simulink model "manual_control_new"  (R2023a)
settings: Solver=FixedStepAuto  StartTime=0.0  StopTime=inf  FixedStep=Ts_slk  RelTol=1e-3  EnableMultiTasking=on
undefined symbols (not defined in the file): dev, IMU_w_b_bias, Main, meas_pole, P0_phth, P0_ps, pwm_output0, Q_phth, q_ps, R_phth, r_ps, Rz, Ts_EKF_integr, Ts_EKF_meas, Ts_slk, x0_phth, x0_ps
libraries: px4Sensorslib x4, px4lib x1, sharedtransform x1
(part 1 of 2)
settings Model: ExtModeTrigDuration=10  Creator=ArriGE66  LastModifiedBy=User
settings SolverCC: PositivePriorityOrder=on
settings OptimizationCC: EnhancedBackFolding=on  PassReuseOutputArgsAs=Individual arguments  ZeroExternalMemoryAtStartup=off  ZeroInternalMemoryAtStartup=off  MaxStackSize=64  OptimizeBlockOrder=speed  DifferentSizesBufferReuse=on  OptimizationCustomize=off  EfficientTunableParamExpr=on
settings DebuggingCC: ParameterTunabilityLossMsg=error
settings HardwareCC: ProdBitPerPointer=32  ProdBitPerSizeT=32  ProdBitPerPtrDiffT=32  ProdLargestAtomicInteger=Long  ProdLargestAtomicFloat=Double  ProdWordSize=32  ProdLongLongMode=on  ProdHWDeviceType=ARM Compatible->ARM Cortex
settings SFSimCC: MATLABDynamicMemAlloc=off  SimTargetLang=C++
settings RTWCC: Description=Embedded Coder  SystemTargetFile=ert.tlc  HardwareBoard=PX4 Cube Orange  TLCOptions="-aInlineSetEventsForThisBaseRateFcn=TLC_FALSE -aSuppressMultiTaskScheduler=TLC_FALSE  -aRateBasedStepFcn=0"  TemplateMakefile=ert_default_tmf  Toolchain=GNU Tools for PX4 Autopilots  TargetLang=C++
settings CodeAppCC: ForceParamTrailComments=on  IgnoreCustomStorageClasses=off  OperatorAnnotations=on  SimulinkDataObjDesc=on  SFDataObjDesc=on  InsertBlockDesc=on
settings ERTTargetCC: ExtModeTransport=3  ExtModeStaticAlloc=on  ExtModeStaticAllocSize=1024  ExtModeMexFile=ext_xcp  ExtModeIntrfLevel=Level2 - Open

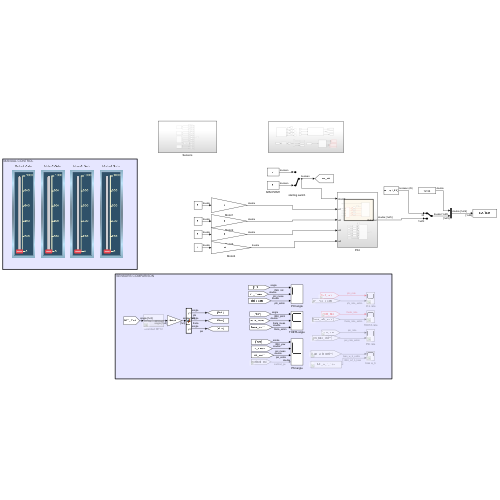
[thumbnail: Simulink's stored preview of the top-level diagram]
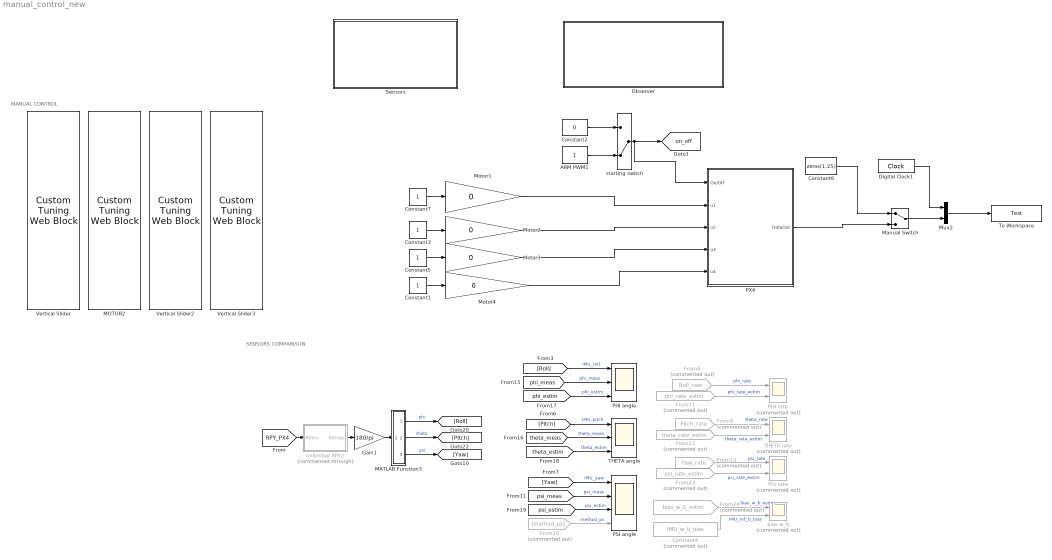
== system manual_control_new ==
  note: SENSORS COMPARISON
  note: MANUAL CONTROL
  ARM PWM1 : Constant  OutDataTypeStr=boolean  SampleTime=Ts_slk
  Constant{1,3,5,7} (4 alike) : Constant  SampleTime=Ts_slk
  Constant2 : Constant  Value=0  OutDataTypeStr=boolean  SampleTime=Ts_slk
  Constant4 : Constant  Commented=on  Value=IMU_w_b_bias
  Constant6 : Constant  Value=zeros(1,25)  OutDataTypeStr=boolean
  Digital Clock1 : DigitalClock  SampleTime=Ts_slk
  From12 : From  Commented=on  GotoTag=Yaw_rate  TagVisibility=global
  From20 : From  Commented=on  GotoTag=method_ps
  From21 : From  Commented=on  GotoTag=phi_rate_estim
  From22 : From  Commented=on  GotoTag=theta_rate_estim
  From23 : From  Commented=on  GotoTag=psi_rate_estim
  From24 : From  Commented=on  GotoTag=bias_w_b_estim
  From8 : From  Commented=on  GotoTag=Roll_rate  TagVisibility=global
  From9 : From  Commented=on  GotoTag=Pitch_rate  TagVisibility=global
  Gain1 : Gain  Gain=180/pi
  MATLAB Function3 : MATLAB Function  TreatAsAtomicUnit=on
  MOTOR2 : CustomTuningWebBlock  ShowInitialText=on  Configuration="{\"components\":[{\"name\":\"LinearScaleComponent\",\"settings\":{\"bounds\":{\"max\":1000,\"min\":0,\"tickInterval\":\"auto\"},\"internalTickHeightScaleFactor\":0.5,\"labelColor\":[255,255,200],\"labelFont\":{\"font\":\"Arial\",\"fontSize\":12},\"labelOffset\":0.05,\"labelTransparency\":1,\"needleImage\":{\"size\":[596,842],\"src\":\"data:image\\/svg+xml;base64,PD94bWwgdmVyc2lvbj0iMS4wIiBlbmNvZGluZz0idXRmLTgiPz4NCjwhLS0gR2VuZXJhdG9yOiBBZG9iZSBJbGx1c3RyYXRvciAyNS4wLjAsIFNWRyBFeHBvcnQgUGx1Zy1JbiAuIFNWRyBWZXJzaW9uOiA2LjAwIEJ1aWxkIDApICAtLT4NCjxzdmcgdmVyc2lvbj0iMS4xIg0KCSBpZD0ic3ZnOCIgeG1sbnM6Y2M9Imh0dHA6Ly9jcmVhdGl2ZWNvbW1vbnMub3JnL25zIyIgeG1sbnM6ZGM9Imh0dHA6Ly9wdXJsLm9yZy9kYy9lbGVtZW50cy8xLjEvIiB4bWxuczppbmtzY2FwZT0iaHR0cDovL3d3dy5pbmtzY2FwZS5vcmcvbmFtZXNw ...(+2420 chars)\",\"srcOrientation\":\"horizontal\"},\"needleOffset\":[0.0642123287671233,-0.8044596912521441],\"needleSize\":{\"height\":0.07668067226890757,\"width\":0.4337797619047619},\"position\":[0.03623949579831933,0.2829861111111111,0.6088789682539683,0.9196428571428571],\"referencePoint\":\"auto\",\"scaleColors\":[],\"scaleColorsSize\":0.2,\"scaleDirection\":\"BT\",\"showLabels\":1,\"showMinorTicks\":0,\"showSpanLine\":1,\"showTicks\":1,\"tickColor\":[252,252,197],\"tickTransparency\":1,\"valueBarColor\":[0,114,189],\"valueBarOffset\":-0.27,\"valueBarSize\":0.1,\"valueBarTransparency\":1}},{\"name\":\"BackgroundImageComponent\",\"settings\":{\"image\":{\"size\":[380,101],\"src\":\"data:image\\/svg+xml;base64,PHN2ZyB4bWxucz0iaHR0cDovL3d3dy53My5vcmcvMjAwMC9zdmciIHhtbG5zOnhsaW5rPSJodHRwOi8vd3d3LnczLm9yZy8xOTk5L3hsaW5rIiB2aWV3Qm94PSIwIDAgMzgwIDEwMSI+PGRlZnM+PHN0eWxlPi5jbHMtMXtmaWxsOiMwMDJiNDI7fS5jbHMtMntmaWxsOiM0MjcwODI7fS5jbHMtM3tmaWxsOnVybCgjcmFkaWFsLWdyYWRpZW50KTt9LmNscy00e2ZpbGw6I2M4YzhjODtzdHJva2U6IzAwMDt9PC9zdHlsZT48cmFkaWFsR3JhZGllbnQgaWQ9InJhZGlhbC1ncmFkaWVudCIgY3g9IjE5MCIgY3k9IjUwLjUiIHI9IjI2OS4yMSIgZ3JhZGllbnRVbml0cz0idXNlclNwYWNlT25Vc2UiPjxzdG9wIG9mZnNldD0iMC4wMSIgc3RvcC1jb2xvcj0iIzNlNGY1OCIvPjxzdG9wIG9mZnNldD0iMC4wNiIgc3RvcC1jb2xvcj0iIzQ0NTc2MSIvPjxzdG9wIG9mZnNldD0iMC4xNSIgc3RvcC1jb2xvcj0iIzU1NmE3NiIvPjxzdG9wIG9mZnNldD0iMC4yNSIgc3RvcC1jb2xvcj0iIzZkODg5NSIvPjxzdG9wIG9mZnNldD0iMC4zOCIgc3RvcC1jb2xvcj0iIzhmYjJjMyIvPjxzdG9wIG9mZnNldD0iMC41MiIgc3RvcC1jb2xvcj0iI2I2ZTRmYSIvPjxzdG9wIG9mZnNldD0iMSIgc3RvcC1jb2xvcj0iIzE1NDY1NyIvPjwvcmFkaWFsR3JhZGllbnQ+PC9kZWZzPjxnIGlkPSJmcmFtZSI+PGcgaWQ9IkxheWVyXzIiIGRhdGEtbmFtZT0iTGF5ZXIgMiI+PGcgaWQ9IkxheWVyXzEtMiIgZGF0YS1uYW1lPSJMYXllciAxLTIiPjxyZWN0IGlkPSJyZWN0MTAzNiIgY2xhc3M9ImNscy0xIiB4PSIxMSIgeT0iMTEiIHdpZHRoPSIzNTgiIGhlaWdodD0iNzkiLz48cGF0aCBpZD0icGF0aDEwMzgiIGNsYXNzPSJjbHMtMiIgZD0iTTgsOFY5M0gzNzJWOFpNMzY5LDkwSDExVjExSDM2OVoiLz48cGF0aCBpZD0icGF0aDEwNDAiIGNsYXNzPSJjbHMtMyIgZD0iTTAsMFYxMDFIMzgwVjBaTTM3Miw5M0g4VjhIMzcyWiIvPjwvZz48L2c+PC9nPjxnIGlkPSJ0cmFjayI+PHBhdGggaWQ9InJlY3QxNjExIiBjbGFzcz0iY2xzLTQiIGQ9Ik0zMy4zNywyNi41OUgzNDYuNjNjNCwwLDcuMjUsMi42LDcuMjUsNS44MWgwYzAsMy4yMS0zLjI1LDUuODItNy4yNSw1LjgySDMzLjM3Yy00LDAtNy4yNS0yLjYxLTcuMjUtNS44MmgwQzI2LjEyLDI5LjE5LDI5LjM3LDI2LjU5LDMzLjM3LDI2LjU5WiIvPjwvZz48L3N2Zz4=\",\"srcOrientation\":\"horizontal\"},\"position\":[0,0,1,1],\"scaleMode\":\"0\"}},{\"name\":\"ForegroundImageComponent\",\"settings\":{\"image\":{\"size\":[0,0],\"src\":\"default\",\"srcOrientation\":[]},\"isForeground\":1,\"position\":[0,0,1,1],\"scaleMode\":\"0\"}}],\"settings\":{\"BindingType\":\"param\",\"aspectRatio\":3.7777777777777777,\"backgroundColor\":[0,0,0,\"1\"],\"backgroundOffset\":0,\"backgroundOpacity\":1,\"fixedAspectRatio\":\"on\",\"foregroundColor\":[252,252,196],\"orientation\":\"vertical\",\"showBackgroundColor\":false,\"value\":0,\"version\":\"R2023a\"},\"type\":\"LinearGauge\"}"
  Manual Switch : ManualSwitch
  Motor{1..4} (4 alike) : Gain  Gain=0
  Mux2 : Mux  Inputs=2
  Observer : Subsystem
  PHI angle : Scope  NumInputPorts=3
  PHI rate : Scope  Commented=on  NumInputPorts=2
  PSI angle : Scope  NumInputPorts=4
  PSI rate : Scope  Commented=on  NumInputPorts=2
  PX4 : Subsystem
  Sensors : Subsystem
  THETA angle : Scope  NumInputPorts=3
  THETA rate : Scope  Commented=on  NumInputPorts=2
  To Workspace : ToWorkspace  VariableName=Test  SampleTime=Ts_slk
      settings: Save2DSignal=2-D array (concatenate along first dimension)
  Vertical Slider : CustomTuningWebBlock  ShowInitialText=on  Configuration="{\"components\":[{\"name\":\"LinearScaleComponent\",\"settings\":{\"bounds\":{\"max\":1000,\"min\":0,\"tickInterval\":\"auto\"},\"internalTickHeightScaleFactor\":0.5,\"labelColor\":[255,255,200],\"labelFont\":{\"font\":\"Arial\",\"fontSize\":12},\"labelOffset\":0.05,\"labelTransparency\":1,\"needleImage\":{\"size\":[596,842],\"src\":\"data:image\\/svg+xml;base64,PD94bWwgdmVyc2lvbj0iMS4wIiBlbmNvZGluZz0idXRmLTgiPz4NCjwhLS0gR2VuZXJhdG9yOiBBZG9iZSBJbGx1c3RyYXRvciAyNS4wLjAsIFNWRyBFeHBvcnQgUGx1Zy1JbiAuIFNWRyBWZXJzaW9uOiA2LjAwIEJ1aWxkIDApICAtLT4NCjxzdmcgdmVyc2lvbj0iMS4xIg0KCSBpZD0ic3ZnOCIgeG1sbnM6Y2M9Imh0dHA6Ly9jcmVhdGl2ZWNvbW1vbnMub3JnL25zIyIgeG1sbnM6ZGM9Imh0dHA6Ly9wdXJsLm9yZy9kYy9lbGVtZW50cy8xLjEvIiB4bWxuczppbmtzY2FwZT0iaHR0cDovL3d3dy5pbmtzY2FwZS5vcmcvbmFtZXNw ...(+2420 chars)\",\"srcOrientation\":\"horizontal\"},\"needleOffset\":[0.0642123287671233,-0.8044596912521441],\"needleSize\":{\"height\":0.07668067226890757,\"width\":0.4337797619047619},\"position\":[0.03623949579831933,0.2829861111111111,0.6088789682539683,0.9196428571428571],\"referencePoint\":\"auto\",\"scaleColors\":[],\"scaleColorsSize\":0.2,\"scaleDirection\":\"BT\",\"showLabels\":1,\"showMinorTicks\":0,\"showSpanLine\":1,\"showTicks\":1,\"tickColor\":[252,252,197],\"tickTransparency\":1,\"valueBarColor\":[0,114,189],\"valueBarOffset\":-0.27,\"valueBarSize\":0.1,\"valueBarTransparency\":1}},{\"name\":\"BackgroundImageComponent\",\"settings\":{\"image\":{\"size\":[380,101],\"src\":\"data:image\\/svg+xml;base64,PHN2ZyB4bWxucz0iaHR0cDovL3d3dy53My5vcmcvMjAwMC9zdmciIHhtbG5zOnhsaW5rPSJodHRwOi8vd3d3LnczLm9yZy8xOTk5L3hsaW5rIiB2aWV3Qm94PSIwIDAgMzgwIDEwMSI+PGRlZnM+PHN0eWxlPi5jbHMtMXtmaWxsOiMwMDJiNDI7fS5jbHMtMntmaWxsOiM0MjcwODI7fS5jbHMtM3tmaWxsOnVybCgjcmFkaWFsLWdyYWRpZW50KTt9LmNscy00e2ZpbGw6I2M4YzhjODtzdHJva2U6IzAwMDt9PC9zdHlsZT48cmFkaWFsR3JhZGllbnQgaWQ9InJhZGlhbC1ncmFkaWVudCIgY3g9IjE5MCIgY3k9IjUwLjUiIHI9IjI2OS4yMSIgZ3JhZGllbnRVbml0cz0idXNlclNwYWNlT25Vc2UiPjxzdG9wIG9mZnNldD0iMC4wMSIgc3RvcC1jb2xvcj0iIzNlNGY1OCIvPjxzdG9wIG9mZnNldD0iMC4wNiIgc3RvcC1jb2xvcj0iIzQ0NTc2MSIvPjxzdG9wIG9mZnNldD0iMC4xNSIgc3RvcC1jb2xvcj0iIzU1NmE3NiIvPjxzdG9wIG9mZnNldD0iMC4yNSIgc3RvcC1jb2xvcj0iIzZkODg5NSIvPjxzdG9wIG9mZnNldD0iMC4zOCIgc3RvcC1jb2xvcj0iIzhmYjJjMyIvPjxzdG9wIG9mZnNldD0iMC41MiIgc3RvcC1jb2xvcj0iI2I2ZTRmYSIvPjxzdG9wIG9mZnNldD0iMSIgc3RvcC1jb2xvcj0iIzE1NDY1NyIvPjwvcmFkaWFsR3JhZGllbnQ+PC9kZWZzPjxnIGlkPSJmcmFtZSI+PGcgaWQ9IkxheWVyXzIiIGRhdGEtbmFtZT0iTGF5ZXIgMiI+PGcgaWQ9IkxheWVyXzEtMiIgZGF0YS1uYW1lPSJMYXllciAxLTIiPjxyZWN0IGlkPSJyZWN0MTAzNiIgY2xhc3M9ImNscy0xIiB4PSIxMSIgeT0iMTEiIHdpZHRoPSIzNTgiIGhlaWdodD0iNzkiLz48cGF0aCBpZD0icGF0aDEwMzgiIGNsYXNzPSJjbHMtMiIgZD0iTTgsOFY5M0gzNzJWOFpNMzY5LDkwSDExVjExSDM2OVoiLz48cGF0aCBpZD0icGF0aDEwNDAiIGNsYXNzPSJjbHMtMyIgZD0iTTAsMFYxMDFIMzgwVjBaTTM3Miw5M0g4VjhIMzcyWiIvPjwvZz48L2c+PC9nPjxnIGlkPSJ0cmFjayI+PHBhdGggaWQ9InJlY3QxNjExIiBjbGFzcz0iY2xzLTQiIGQ9Ik0zMy4zNywyNi41OUgzNDYuNjNjNCwwLDcuMjUsMi42LDcuMjUsNS44MWgwYzAsMy4yMS0zLjI1LDUuODItNy4yNSw1LjgySDMzLjM3Yy00LDAtNy4yNS0yLjYxLTcuMjUtNS44MmgwQzI2LjEyLDI5LjE5LDI5LjM3LDI2LjU5LDMzLjM3LDI2LjU5WiIvPjwvZz48L3N2Zz4=\",\"srcOrientation\":\"horizontal\"},\"position\":[0,0,1,1],\"scaleMode\":\"0\"}},{\"name\":\"ForegroundImageComponent\",\"settings\":{\"image\":{\"size\":[0,0],\"src\":\"default\",\"srcOrientation\":[]},\"isForeground\":1,\"position\":[0,0,1,1],\"scaleMode\":\"0\"}}],\"settings\":{\"BindingType\":\"param\",\"aspectRatio\":3.7777777777777777,\"backgroundColor\":[0,0,0,\"1\"],\"backgroundOffset\":0,\"backgroundOpacity\":1,\"fixedAspectRatio\":\"on\",\"foregroundColor\":[252,252,196],\"orientation\":\"vertical\",\"showBackgroundColor\":false,\"value\":0,\"version\":\"R2023a\"},\"type\":\"LinearGauge\"}"
  Vertical Slider2 : CustomTuningWebBlock  ShowInitialText=on  Configuration="{\"components\":[{\"name\":\"LinearScaleComponent\",\"settings\":{\"bounds\":{\"max\":1000,\"min\":0,\"tickInterval\":\"auto\"},\"internalTickHeightScaleFactor\":0.5,\"labelColor\":[255,255,200],\"labelFont\":{\"font\":\"Arial\",\"fontSize\":12},\"labelOffset\":0.05,\"labelTransparency\":1,\"needleImage\":{\"size\":[596,842],\"src\":\"data:image\\/svg+xml;base64,PD94bWwgdmVyc2lvbj0iMS4wIiBlbmNvZGluZz0idXRmLTgiPz4NCjwhLS0gR2VuZXJhdG9yOiBBZG9iZSBJbGx1c3RyYXRvciAyNS4wLjAsIFNWRyBFeHBvcnQgUGx1Zy1JbiAuIFNWRyBWZXJzaW9uOiA2LjAwIEJ1aWxkIDApICAtLT4NCjxzdmcgdmVyc2lvbj0iMS4xIg0KCSBpZD0ic3ZnOCIgeG1sbnM6Y2M9Imh0dHA6Ly9jcmVhdGl2ZWNvbW1vbnMub3JnL25zIyIgeG1sbnM6ZGM9Imh0dHA6Ly9wdXJsLm9yZy9kYy9lbGVtZW50cy8xLjEvIiB4bWxuczppbmtzY2FwZT0iaHR0cDovL3d3dy5pbmtzY2FwZS5vcmcvbmFtZXNw ...(+2420 chars)\",\"srcOrientation\":\"horizontal\"},\"needleOffset\":[0.0642123287671233,-0.8044596912521441],\"needleSize\":{\"height\":0.07668067226890757,\"width\":0.4337797619047619},\"position\":[0.03623949579831933,0.2829861111111111,0.6088789682539683,0.9196428571428571],\"referencePoint\":\"auto\",\"scaleColors\":[],\"scaleColorsSize\":0.2,\"scaleDirection\":\"BT\",\"showLabels\":1,\"showMinorTicks\":0,\"showSpanLine\":1,\"showTicks\":1,\"tickColor\":[252,252,197],\"tickTransparency\":1,\"valueBarColor\":[0,114,189],\"valueBarOffset\":-0.27,\"valueBarSize\":0.1,\"valueBarTransparency\":1}},{\"name\":\"BackgroundImageComponent\",\"settings\":{\"image\":{\"size\":[380,101],\"src\":\"data:image\\/svg+xml;base64,PHN2ZyB4bWxucz0iaHR0cDovL3d3dy53My5vcmcvMjAwMC9zdmciIHhtbG5zOnhsaW5rPSJodHRwOi8vd3d3LnczLm9yZy8xOTk5L3hsaW5rIiB2aWV3Qm94PSIwIDAgMzgwIDEwMSI+PGRlZnM+PHN0eWxlPi5jbHMtMXtmaWxsOiMwMDJiNDI7fS5jbHMtMntmaWxsOiM0MjcwODI7fS5jbHMtM3tmaWxsOnVybCgjcmFkaWFsLWdyYWRpZW50KTt9LmNscy00e2ZpbGw6I2M4YzhjODtzdHJva2U6IzAwMDt9PC9zdHlsZT48cmFkaWFsR3JhZGllbnQgaWQ9InJhZGlhbC1ncmFkaWVudCIgY3g9IjE5MCIgY3k9IjUwLjUiIHI9IjI2OS4yMSIgZ3JhZGllbnRVbml0cz0idXNlclNwYWNlT25Vc2UiPjxzdG9wIG9mZnNldD0iMC4wMSIgc3RvcC1jb2xvcj0iIzNlNGY1OCIvPjxzdG9wIG9mZnNldD0iMC4wNiIgc3RvcC1jb2xvcj0iIzQ0NTc2MSIvPjxzdG9wIG9mZnNldD0iMC4xNSIgc3RvcC1jb2xvcj0iIzU1NmE3NiIvPjxzdG9wIG9mZnNldD0iMC4yNSIgc3RvcC1jb2xvcj0iIzZkODg5NSIvPjxzdG9wIG9mZnNldD0iMC4zOCIgc3RvcC1jb2xvcj0iIzhmYjJjMyIvPjxzdG9wIG9mZnNldD0iMC41MiIgc3RvcC1jb2xvcj0iI2I2ZTRmYSIvPjxzdG9wIG9mZnNldD0iMSIgc3RvcC1jb2xvcj0iIzE1NDY1NyIvPjwvcmFkaWFsR3JhZGllbnQ+PC9kZWZzPjxnIGlkPSJmcmFtZSI+PGcgaWQ9IkxheWVyXzIiIGRhdGEtbmFtZT0iTGF5ZXIgMiI+PGcgaWQ9IkxheWVyXzEtMiIgZGF0YS1uYW1lPSJMYXllciAxLTIiPjxyZWN0IGlkPSJyZWN0MTAzNiIgY2xhc3M9ImNscy0xIiB4PSIxMSIgeT0iMTEiIHdpZHRoPSIzNTgiIGhlaWdodD0iNzkiLz48cGF0aCBpZD0icGF0aDEwMzgiIGNsYXNzPSJjbHMtMiIgZD0iTTgsOFY5M0gzNzJWOFpNMzY5LDkwSDExVjExSDM2OVoiLz48cGF0aCBpZD0icGF0aDEwNDAiIGNsYXNzPSJjbHMtMyIgZD0iTTAsMFYxMDFIMzgwVjBaTTM3Miw5M0g4VjhIMzcyWiIvPjwvZz48L2c+PC9nPjxnIGlkPSJ0cmFjayI+PHBhdGggaWQ9InJlY3QxNjExIiBjbGFzcz0iY2xzLTQiIGQ9Ik0zMy4zNywyNi41OUgzNDYuNjNjNCwwLDcuMjUsMi42LDcuMjUsNS44MWgwYzAsMy4yMS0zLjI1LDUuODItNy4yNSw1LjgySDMzLjM3Yy00LDAtNy4yNS0yLjYxLTcuMjUtNS44MmgwQzI2LjEyLDI5LjE5LDI5LjM3LDI2LjU5LDMzLjM3LDI2LjU5WiIvPjwvZz48L3N2Zz4=\",\"srcOrientation\":\"horizontal\"},\"position\":[0,0,1,1],\"scaleMode\":\"0\"}},{\"name\":\"ForegroundImageComponent\",\"settings\":{\"image\":{\"size\":[0,0],\"src\":\"default\",\"srcOrientation\":[]},\"isForeground\":1,\"position\":[0,0,1,1],\"scaleMode\":\"0\"}}],\"settings\":{\"BindingType\":\"param\",\"aspectRatio\":3.7777777777777777,\"backgroundColor\":[0,0,0,\"1\"],\"backgroundOffset\":0,\"backgroundOpacity\":1,\"fixedAspectRatio\":\"on\",\"foregroundColor\":[252,252,196],\"orientation\":\"vertical\",\"showBackgroundColor\":false,\"value\":0,\"version\":\"R2023a\"},\"type\":\"LinearGauge\"}"
  Vertical Slider3 : CustomTuningWebBlock  ShowInitialText=on  Configuration="{\"components\":[{\"name\":\"LinearScaleComponent\",\"settings\":{\"bounds\":{\"max\":1000,\"min\":0,\"tickInterval\":\"auto\"},\"internalTickHeightScaleFactor\":0.5,\"labelColor\":[255,255,200],\"labelFont\":{\"font\":\"Arial\",\"fontSize\":12},\"labelOffset\":0.05,\"labelTransparency\":1,\"needleImage\":{\"size\":[596,842],\"src\":\"data:image\\/svg+xml;base64,PD94bWwgdmVyc2lvbj0iMS4wIiBlbmNvZGluZz0idXRmLTgiPz4NCjwhLS0gR2VuZXJhdG9yOiBBZG9iZSBJbGx1c3RyYXRvciAyNS4wLjAsIFNWRyBFeHBvcnQgUGx1Zy1JbiAuIFNWRyBWZXJzaW9uOiA2LjAwIEJ1aWxkIDApICAtLT4NCjxzdmcgdmVyc2lvbj0iMS4xIg0KCSBpZD0ic3ZnOCIgeG1sbnM6Y2M9Imh0dHA6Ly9jcmVhdGl2ZWNvbW1vbnMub3JnL25zIyIgeG1sbnM6ZGM9Imh0dHA6Ly9wdXJsLm9yZy9kYy9lbGVtZW50cy8xLjEvIiB4bWxuczppbmtzY2FwZT0iaHR0cDovL3d3dy5pbmtzY2FwZS5vcmcvbmFtZXNw ...(+2420 chars)\",\"srcOrientation\":\"horizontal\"},\"needleOffset\":[0.0642123287671233,-0.8044596912521441],\"needleSize\":{\"height\":0.07668067226890757,\"width\":0.4337797619047619},\"position\":[0.03623949579831933,0.2829861111111111,0.6088789682539683,0.9196428571428571],\"referencePoint\":\"auto\",\"scaleColors\":[],\"scaleColorsSize\":0.2,\"scaleDirection\":\"BT\",\"showLabels\":1,\"showMinorTicks\":0,\"showSpanLine\":1,\"showTicks\":1,\"tickColor\":[252,252,197],\"tickTransparency\":1,\"valueBarColor\":[0,114,189],\"valueBarOffset\":-0.27,\"valueBarSize\":0.1,\"valueBarTransparency\":1}},{\"name\":\"BackgroundImageComponent\",\"settings\":{\"image\":{\"size\":[380,101],\"src\":\"data:image\\/svg+xml;base64,PHN2ZyB4bWxucz0iaHR0cDovL3d3dy53My5vcmcvMjAwMC9zdmciIHhtbG5zOnhsaW5rPSJodHRwOi8vd3d3LnczLm9yZy8xOTk5L3hsaW5rIiB2aWV3Qm94PSIwIDAgMzgwIDEwMSI+PGRlZnM+PHN0eWxlPi5jbHMtMXtmaWxsOiMwMDJiNDI7fS5jbHMtMntmaWxsOiM0MjcwODI7fS5jbHMtM3tmaWxsOnVybCgjcmFkaWFsLWdyYWRpZW50KTt9LmNscy00e2ZpbGw6I2M4YzhjODtzdHJva2U6IzAwMDt9PC9zdHlsZT48cmFkaWFsR3JhZGllbnQgaWQ9InJhZGlhbC1ncmFkaWVudCIgY3g9IjE5MCIgY3k9IjUwLjUiIHI9IjI2OS4yMSIgZ3JhZGllbnRVbml0cz0idXNlclNwYWNlT25Vc2UiPjxzdG9wIG9mZnNldD0iMC4wMSIgc3RvcC1jb2xvcj0iIzNlNGY1OCIvPjxzdG9wIG9mZnNldD0iMC4wNiIgc3RvcC1jb2xvcj0iIzQ0NTc2MSIvPjxzdG9wIG9mZnNldD0iMC4xNSIgc3RvcC1jb2xvcj0iIzU1NmE3NiIvPjxzdG9wIG9mZnNldD0iMC4yNSIgc3RvcC1jb2xvcj0iIzZkODg5NSIvPjxzdG9wIG9mZnNldD0iMC4zOCIgc3RvcC1jb2xvcj0iIzhmYjJjMyIvPjxzdG9wIG9mZnNldD0iMC41MiIgc3RvcC1jb2xvcj0iI2I2ZTRmYSIvPjxzdG9wIG9mZnNldD0iMSIgc3RvcC1jb2xvcj0iIzE1NDY1NyIvPjwvcmFkaWFsR3JhZGllbnQ+PC9kZWZzPjxnIGlkPSJmcmFtZSI+PGcgaWQ9IkxheWVyXzIiIGRhdGEtbmFtZT0iTGF5ZXIgMiI+PGcgaWQ9IkxheWVyXzEtMiIgZGF0YS1uYW1lPSJMYXllciAxLTIiPjxyZWN0IGlkPSJyZWN0MTAzNiIgY2xhc3M9ImNscy0xIiB4PSIxMSIgeT0iMTEiIHdpZHRoPSIzNTgiIGhlaWdodD0iNzkiLz48cGF0aCBpZD0icGF0aDEwMzgiIGNsYXNzPSJjbHMtMiIgZD0iTTgsOFY5M0gzNzJWOFpNMzY5LDkwSDExVjExSDM2OVoiLz48cGF0aCBpZD0icGF0aDEwNDAiIGNsYXNzPSJjbHMtMyIgZD0iTTAsMFYxMDFIMzgwVjBaTTM3Miw5M0g4VjhIMzcyWiIvPjwvZz48L2c+PC9nPjxnIGlkPSJ0cmFjayI+PHBhdGggaWQ9InJlY3QxNjExIiBjbGFzcz0iY2xzLTQiIGQ9Ik0zMy4zNywyNi41OUgzNDYuNjNjNCwwLDcuMjUsMi42LDcuMjUsNS44MWgwYzAsMy4yMS0zLjI1LDUuODItNy4yNSw1LjgySDMzLjM3Yy00LDAtNy4yNS0yLjYxLTcuMjUtNS44MmgwQzI2LjEyLDI5LjE5LDI5LjM3LDI2LjU5LDMzLjM3LDI2LjU5WiIvPjwvZz48L3N2Zz4=\",\"srcOrientation\":\"horizontal\"},\"position\":[0,0,1,1],\"scaleMode\":\"0\"}},{\"name\":\"ForegroundImageComponent\",\"settings\":{\"image\":{\"size\":[0,0],\"src\":\"default\",\"srcOrientation\":[]},\"isForeground\":1,\"position\":[0,0,1,1],\"scaleMode\":\"0\"}}],\"settings\":{\"BindingType\":\"param\",\"aspectRatio\":3.7777777777777777,\"backgroundColor\":[0,0,0,\"1\"],\"backgroundOffset\":0,\"backgroundOpacity\":1,\"fixedAspectRatio\":\"on\",\"foregroundColor\":[252,252,196],\"orientation\":\"vertical\",\"showBackgroundColor\":false,\"value\":0,\"version\":\"R2023a\"},\"type\":\"LinearGauge\"}"
  bias w_b : Scope  Commented=on  NumInputPorts=2
  starting switch : ManualSwitch  CurrentSetting=0
  unlimited RPY2 : Subsystem  Commented=through
  tag scope: on_off=global
  wires:
  Motor2/1 -> PX4/3(u2)
  ARM PWM1/1 -> starting switch/2
  Constant2/1 -> starting switch/1
  starting switch/1 -> PX4/1(On/Off), [on_off]
  Motor1/1 -> PX4/2(u1)
  Motor4/1 -> PX4/5(u4)
  Motor3/1 -> PX4/4(u3)
  [phi_estim] -> PHI angle/3  "phi_estim"
  From8/1 -> PHI rate/1  "phi_rate"
  [RPY_PX4] -> unlimited RPY2/1(RPYin)
  MATLAB Function3/3(y3) -> [Yaw]  "psi"
  MATLAB Function3/1(y1) -> [Roll]  "phi"
  From12/1 -> PSI rate/1  "psi_rate"
  From24/1 -> bias w_b/1  "bias_w_b_estim"
  [phi_meas] -> PHI angle/2  "phi_meas"
  [theta_meas] -> THETA angle/2  "theta_meas"
  From9/1 -> THETA rate/1  "theta_rate"
  From21/1 -> PHI rate/2  "phi_rate_estim"
  [Pitch] -> THETA angle/1  "IMU_pitch"
  From20/1 -> PSI angle/4  "method_ps"
  [Yaw] -> PSI angle/1  "IMU_yaw"
  From22/1 -> THETA rate/2  "theta_rate_estim"
  [psi_meas] -> PSI angle/2  "psi_meas"
  MATLAB Function3/2(y2) -> [Pitch]  "theta"
  [psi_estim] -> PSI angle/3  "psi_estim"
  unlimited RPY2/1(RPYout) -> Gain1/1
  [Roll] -> PHI angle/1  "IMU_roll"
  [theta_estim] -> THETA angle/3  "theta_estim"
  Constant4/1 -> bias w_b/2  "IMU_mf_b_bias"
  From23/1 -> PSI rate/2  "psi_rate_estim"
  Gain1/1 -> MATLAB Function3/1(u)
  Mux2/1 -> To Workspace/1
  Digital Clock1/1 -> Mux2/1
  Constant6/1 -> Manual Switch/1
  PX4/1(DataOut) -> Manual Switch/2
  Constant1/1 -> Motor4/1
  Constant3/1 -> Motor2/1
  Constant7/1 -> Motor1/1
  Constant5/1 -> Motor3/1
  Manual Switch/1 -> Mux2/2

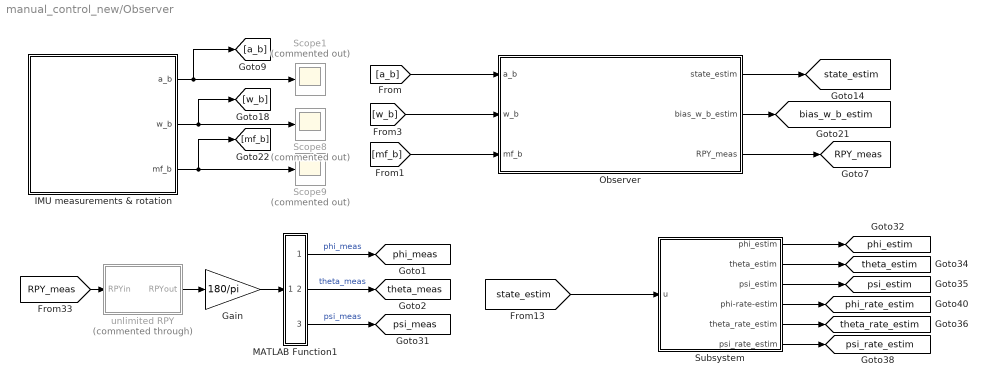
== system manual_control_new/Observer ==
  Gain : Gain  Gain=180/pi
  IMU measurements & rotation : Subsystem
  MATLAB Function1 : MATLAB Function  TreatAsAtomicUnit=on
  Observer : Subsystem
  Scope1 : Scope  Commented=on
  Scope8 : Scope  Commented=on
  Scope9 : Scope  Commented=on
  Subsystem : Subsystem
  unlimited RPY : Subsystem  Commented=through
  tag scope: RPY_meas=global, bias_w_b_estim=global, phi_estim=global, phi_meas=global, phi_rate_estim=global, psi_estim=global, psi_meas=global, psi_rate_estim=global, state_estim=global, theta_estim=global, theta_meas=global, theta_rate_estim=global
  wires:
  MATLAB Function1/1(y1) -> [phi_meas]  "phi_meas"
  [w_b] -> Observer/2(w_b)
  Subsystem/6(psi_rate_estim) -> [psi_rate_estim]
  IMU measurements & rotation/1(a_b) -> [a_b], Scope1/1
  Subsystem/5(theta_rate_estim) -> [theta_rate_estim]
  Observer/2(bias_w_b_estim) -> [bias_w_b_estim]
  Observer/1(state_estim) -> [state_estim]
  [state_estim] -> Subsystem/1(u)
  MATLAB Function1/2(y2) -> [theta_meas]  "theta_meas"
  Observer/3(RPY_meas) -> [RPY_meas]
  [a_b] -> Observer/1(a_b)
  Subsystem/4(phi-rate-estim) -> [phi_rate_estim]
  [RPY_meas] -> unlimited RPY/1(RPYin)
  [mf_b] -> Observer/3(mf_b)
  Subsystem/3(psi_estim) -> [psi_estim]
  unlimited RPY/1(RPYout) -> Gain/1
  Subsystem/2(theta_estim) -> [theta_estim]
  Subsystem/1(phi_estim) -> [phi_estim]
  Gain/1 -> MATLAB Function1/1(u)
  MATLAB Function1/3(y3) -> [psi_meas]  "psi_meas"
  IMU measurements & rotation/3(mf_b) -> [mf_b], Scope9/1
  IMU measurements & rotation/2(w_b) -> [w_b], Scope8/1

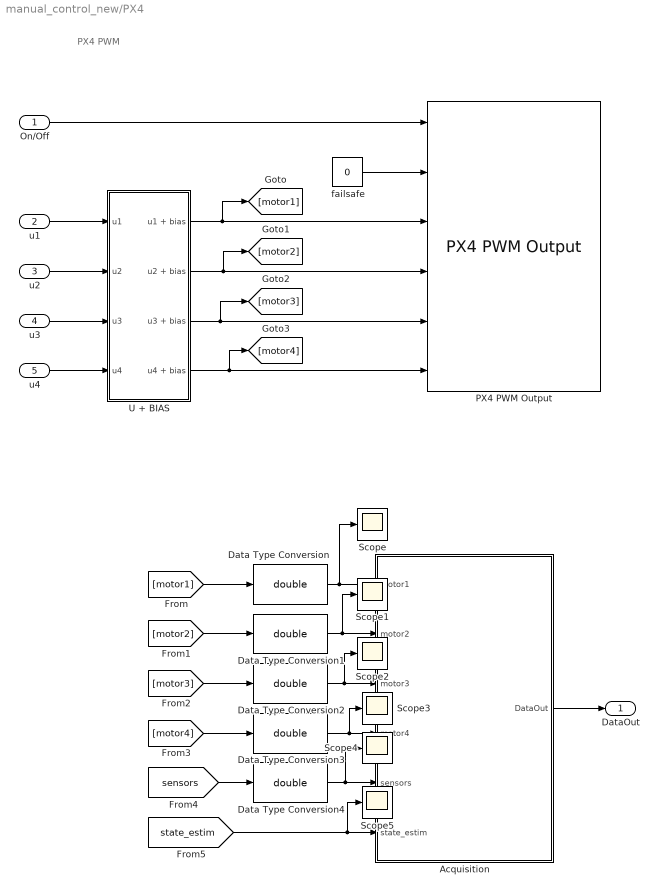
== system manual_control_new/PX4 ==
  note: PX4 PWM
  On/Off : Inport
  u1 : Inport  Port=2
  u2 : Inport  Port=3
  u3 : Inport  Port=4
  u4 : Inport  Port=5
  Acquisition : Subsystem
  Data Type Conversion{,1..4} (5 alike) : DataTypeConversion  OutDataTypeStr=double  RndMeth=Nearest  SaturateOnIntegerOverflow=off
  PX4 PWM Output : px4lib/PX4 PWM Output  pwmDevice=Main (/dev/pwm_output0)  pwmChannel1_=on  pwmChannel2_=on  pwmChannel3_=on  pwmChannel4_=on  pwmChannel5_=off  pwmChannel6_=off  pwmChannel7_=off  pwmChannel8_=off  forceTerminateFailsafe=off  outputErrorStatus=off
  Scope{,1..5} (6 alike) : Scope
  U + BIAS : Subsystem
  failsafe : Constant  Value=0  OutDataTypeStr=boolean  SampleTime=Ts_slk
  DataOut : Outport
  wires:
  On/Off/1 -> PX4 PWM Output/1
  u1/1 -> U + BIAS/1(u1)
  u2/1 -> U + BIAS/2(u2)
  u4/1 -> U + BIAS/4(u4)
  u3/1 -> U + BIAS/3(u3)
  failsafe/1 -> PX4 PWM Output/2
  U + BIAS/1(u1 + bias) -> [motor1], PX4 PWM Output/3
  U + BIAS/2(u2 + bias) -> PX4 PWM Output/4, [motor2]
  U + BIAS/3(u3 + bias) -> PX4 PWM Output/5, [motor3]
  U + BIAS/4(u4 + bias) -> [motor4], PX4 PWM Output/6
  [sensors] -> Data Type Conversion4/1
  [motor1] -> Data Type Conversion/1
  [motor2] -> Data Type Conversion1/1
  [motor3] -> Data Type Conversion2/1
  [motor4] -> Data Type Conversion3/1
  Acquisition/1(DataOut) -> DataOut/1
  Data Type Conversion/1 -> Scope/1, Acquisition/1(motor1)
  Data Type Conversion1/1 -> Scope1/1, Acquisition/2(motor2)
  Data Type Conversion3/1 -> Scope3/1, Acquisition/4(motor4)
  Data Type Conversion4/1 -> Scope4/1, Acquisition/5(sensors)
  Data Type Conversion2/1 -> Scope2/1, Acquisition/3(motor3)
  [state_estim] -> Scope5/1, Acquisition/6(state_estim)

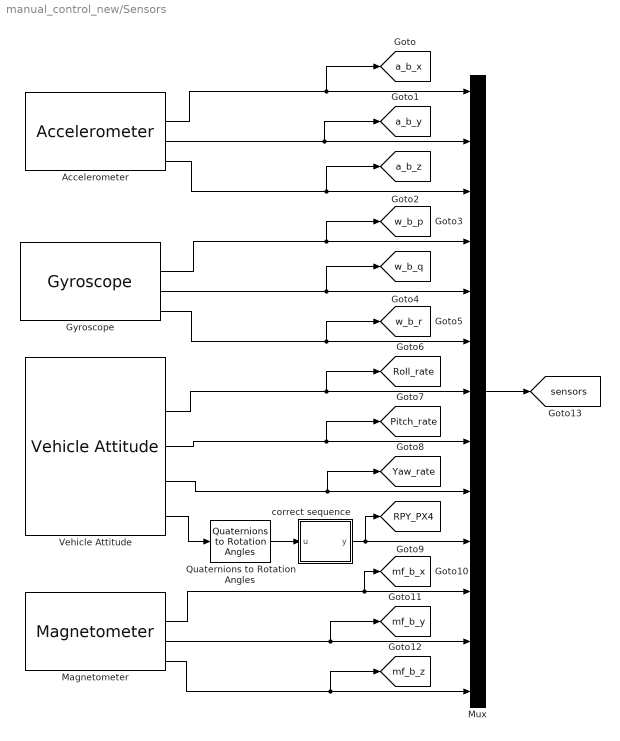
== system manual_control_new/Sensors ==
  Accelerometer : px4Sensorslib/Accelerometer  uorbTimeStamp=off  BlockingMode=off  BlockTimeout=1e-3  sampleTime=Ts_slk
  Gyroscope : px4Sensorslib/Gyroscope  uorbTimeStamp=off  BlockingMode=off  BlockTimeout=1e-3  sampleTime=Ts_slk
  Magnetometer : px4Sensorslib/Magnetometer  uorbTimeStamp=off  BlockingMode=off  BlockTimeout=1e-3  sampleTime=Ts_slk
  Mux : Mux  Inputs=13
  Quaternions to Rotation Angles : sharedtransform/Quaternions to Rotation Angles  rotationOrder=ZYX  aMode=aMode
  Vehicle Attitude : px4Sensorslib/Vehicle Attitude  rollRate=on  pitchRate=on  yawRate=on  quaternion=on  uorbTimeStamp=off  BlockingMode=off  BlockTimeout=0.001  sampleTime=Ts_slk
  correct sequence : MATLAB Function  TreatAsAtomicUnit=on
  tag scope: Pitch_rate=global, RPY_PX4=global, Roll_rate=global, Yaw_rate=global, a_b_x=global, a_b_y=global, a_b_z=global, mf_b_x=global, mf_b_y=global, mf_b_z=global, sensors=global, w_b_p=global, w_b_q=global, w_b_r=global
  wires:
  Vehicle Attitude/3 -> Mux/8, [Pitch_rate]
  Magnetometer/4 -> [mf_b_z], Mux/13
  Quaternions to Rotation Angles/1 -> correct sequence/1(u)
  Gyroscope/2 -> Mux/4, [w_b_p]
  Magnetometer/3 -> [mf_b_y], Mux/12
  Accelerometer/2 -> Mux/1, [a_b_x]
  Vehicle Attitude/4 -> Mux/9, [Yaw_rate]
  Accelerometer/3 -> [a_b_y], Mux/2
  Vehicle Attitude/2 -> Mux/7, [Roll_rate]
  correct sequence/1(y) -> [RPY_PX4], Mux/10
  Gyroscope/4 -> Mux/6, [w_b_r]
  Magnetometer/2 -> Mux/11, [mf_b_x]
  Accelerometer/4 -> Mux/3, [a_b_z]
  Vehicle Attitude/5 -> Quaternions to Rotation Angles/1
  Gyroscope/3 -> Mux/5, [w_b_q]
  Mux/1 -> [sensors]

== system manual_control_new/unlimited RPY2 ==
  RPYin : Inport
  Memory : Memory
  Memory1 : Memory
  unlimited RPY : MATLAB Function  TreatAsAtomicUnit=on
  RPYout : Outport
  wires:
  RPYin/1 -> unlimited RPY/1("RPY ")
  unlimited RPY/1(RPY) -> Memory/1, RPYout/1
  Memory/1 -> unlimited RPY/2(RPY1)
  unlimited RPY/2(init) -> Memory1/1
  Memory1/1 -> unlimited RPY/3("init ")

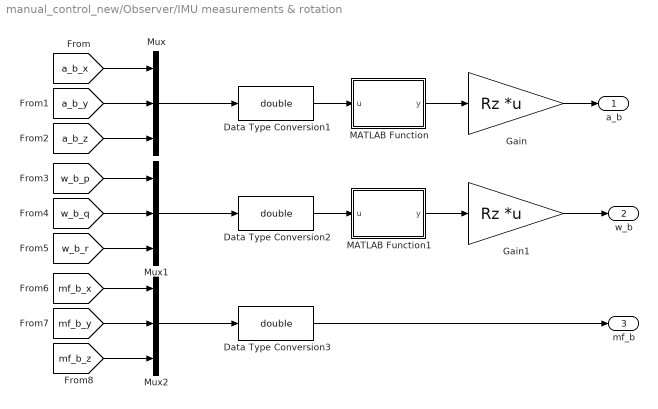
== system manual_control_new/Observer/IMU measurements & rotation ==
  Data Type Conversion1 : DataTypeConversion  OutDataTypeStr=double  SaturateOnIntegerOverflow=off  RndMeth=Floor
  Data Type Conversion2 : DataTypeConversion  OutDataTypeStr=double  SaturateOnIntegerOverflow=off  RndMeth=Floor
  Data Type Conversion3 : DataTypeConversion  OutDataTypeStr=double  SaturateOnIntegerOverflow=off  RndMeth=Floor
  Gain : Gain  Gain=Rz  Multiplication=Matrix(K*u) (u vector)
  Gain1 : Gain  Gain=Rz  Multiplication=Matrix(K*u) (u vector)
  MATLAB Function : MATLAB Function  TreatAsAtomicUnit=on
  MATLAB Function1 : MATLAB Function  TreatAsAtomicUnit=on
  Mux : Mux  Inputs=3
  Mux1 : Mux  Inputs=3
  Mux2 : Mux  Inputs=3
  a_b : Outport
  w_b : Outport  Port=2
  mf_b : Outport  Port=3
  wires:
  [w_b_p] -> Mux1/1
  Data Type Conversion3/1 -> mf_b/1
  Data Type Conversion2/1 -> MATLAB Function1/1(u)
  [mf_b_y] -> Mux2/2
  Mux1/1 -> Data Type Conversion2/1
  Mux/1 -> Data Type Conversion1/1
  [a_b_y] -> Mux/2
  Mux2/1 -> Data Type Conversion3/1
  [w_b_q] -> Mux1/2
  [mf_b_z] -> Mux2/3
  [a_b_z] -> Mux/3
  [a_b_x] -> Mux/1
  [mf_b_x] -> Mux2/1
  [w_b_r] -> Mux1/3
  Gain/1 -> a_b/1
  Data Type Conversion1/1 -> MATLAB Function/1(u)
  MATLAB Function/1(y) -> Gain/1
  MATLAB Function1/1(y) -> Gain1/1
  Gain1/1 -> w_b/1

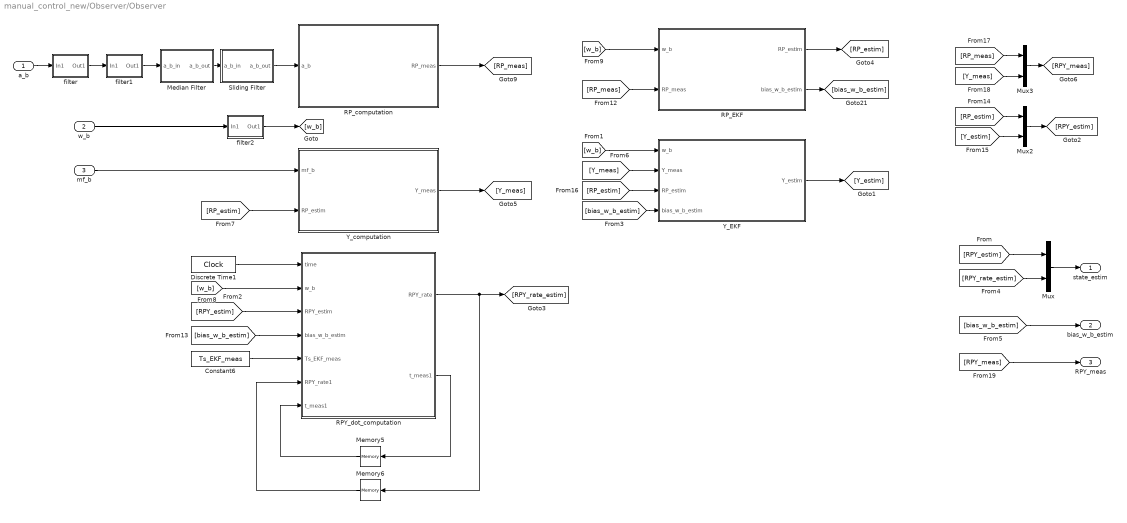
== system manual_control_new/Observer/Observer ==
  a_b : Inport
  w_b : Inport  Port=2
  mf_b : Inport  Port=3
  " filter" : Subsystem  mask{p=5}
      mask prompts: p "pole (p)"
  " filter1" : Subsystem  mask{p=meas_pole}
      mask prompts: p "pole (p)"
  " filter2" : Subsystem  mask{p=meas_pole}
      mask prompts: p "pole (p)"
  Constant6 : Constant  Value=Ts_EKF_meas
  Discrete Time1 : DigitalClock  SampleTime=Ts_slk
  Median Filter : Subsystem
  Memory5 : Memory
  Memory6 : Memory
  Mux : Mux  Inputs=2
  Mux2 : Mux  Inputs=2
  Mux3 : Mux  Inputs=2
  RPY_dot_computation : MATLAB Function  TreatAsAtomicUnit=on
  RP_EKF : Subsystem
  RP_computation : MATLAB Function  TreatAsAtomicUnit=on
  Sliding Filter : Subsystem
  Y_EKF : Subsystem
  Y_computation : MATLAB Function  TreatAsAtomicUnit=on
  state_estim : Outport
  bias_w_b_estim : Outport  Port=2
  RPY_meas : Outport  Port=3
  wires:
  Memory5/1 -> RPY_dot_computation/7("t_meas1 ")
  Discrete Time1/1 -> RPY_dot_computation/1(time)
  RPY_dot_computation/2(t_meas1) -> Memory5/1
  [w_b] -> RPY_dot_computation/2(w_b)
  Memory6/1 -> RPY_dot_computation/6(RPY_rate1)
  RPY_dot_computation/1(RPY_rate) -> Memory6/1, [RPY_rate_estim]
  Constant6/1 -> RPY_dot_computation/5(Ts_EKF_meas)
  [RPY_estim] -> RPY_dot_computation/3(RPY_estim)
  [bias_w_b_estim] -> RPY_dot_computation/4(bias_w_b_estim)
  [RPY_estim] -> Mux/1
  [RPY_rate_estim] -> Mux/2
  Mux/1 -> state_estim/1
  [bias_w_b_estim] -> bias_w_b_estim/1
  [RPY_meas] -> RPY_meas/1
  RP_EKF/2(bias_w_b_estim) -> [bias_w_b_estim]
  [RP_estim] -> Y_computation/2(RP_estim)
  [Y_meas] -> Y_EKF/2(Y_meas)
  Y_computation/1(Y_meas) -> [Y_meas]
  RP_EKF/1(RP_estim) -> [RP_estim]
  [w_b] -> Y_EKF/1(w_b)
  RP_computation/1(RP_meas) -> [RP_meas]
  [RP_meas] -> RP_EKF/2(RP_meas)
  [w_b] -> RP_EKF/1(w_b)
  Y_EKF/1(Y_estim) -> [Y_estim]
  mf_b/1 -> Y_computation/1(mf_b)
  w_b/1 -> " filter2"/1(In1)
  [bias_w_b_estim] -> Y_EKF/4(bias_w_b_estim)
  [RP_estim] -> Mux2/1
  [Y_estim] -> Mux2/2
  Mux2/1 -> [RPY_estim]
  [RP_estim] -> Y_EKF/3(RP_estim)
  [RP_meas] -> Mux3/1
  Mux3/1 -> [RPY_meas]
  [Y_meas] -> Mux3/2
  Sliding Filter/1(a_b_out) -> RP_computation/1(a_b)
  Median Filter/1(a_b_out) -> Sliding Filter/1(a_b_in)
  " filter1"/1(Out1) -> Median Filter/1(a_b_in)
  " filter"/1(Out1) -> " filter1"/1(In1)
  a_b/1 -> " filter"/1(In1)
  " filter2"/1(Out1) -> [w_b]

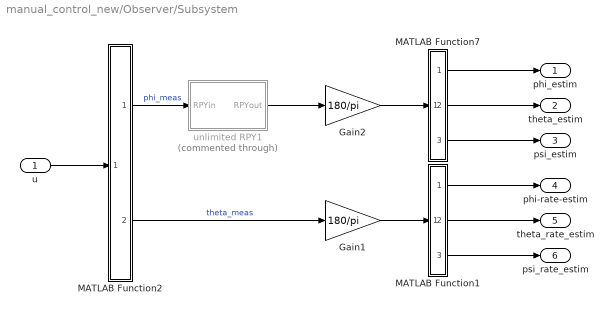
== system manual_control_new/Observer/Subsystem ==
  u : Inport
  Gain1 : Gain  Gain=180/pi
  Gain2 : Gain  Gain=180/pi
  MATLAB Function1 : MATLAB Function  TreatAsAtomicUnit=on
  MATLAB Function2 : MATLAB Function  TreatAsAtomicUnit=on
  MATLAB Function7 : MATLAB Function  TreatAsAtomicUnit=on
  unlimited RPY1 : Subsystem  Commented=through
  phi_estim : Outport
  theta_estim : Outport  Port=2
  psi_estim : Outport  Port=3
  phi-rate-estim : Outport  Port=4
  theta_rate_estim : Outport  Port=5
  psi_rate_estim : Outport  Port=6
  wires:
  u/1 -> MATLAB Function2/1(u)
  MATLAB Function2/2(y2) -> Gain1/1  "theta_meas"
  MATLAB Function2/1(y1) -> unlimited RPY1/1(RPYin)  "phi_meas"
  MATLAB Function7/2(y2) -> theta_estim/1
  MATLAB Function7/1(y1) -> phi_estim/1
  MATLAB Function7/3(y3) -> psi_estim/1
  unlimited RPY1/1(RPYout) -> Gain2/1
  Gain2/1 -> MATLAB Function7/1(u)
  Gain1/1 -> MATLAB Function1/1(u)
  MATLAB Function1/3(y3) -> psi_rate_estim/1
  MATLAB Function1/2(y2) -> theta_rate_estim/1
  MATLAB Function1/1(y1) -> phi-rate-estim/1

== system manual_control_new/Observer/unlimited RPY ==
  RPYin : Inport
  Memory : Memory
  Memory1 : Memory
  unlimited RPY : MATLAB Function  TreatAsAtomicUnit=on
  RPYout : Outport
  wires:
  RPYin/1 -> unlimited RPY/1("RPY ")
  unlimited RPY/1(RPY) -> Memory/1, RPYout/1
  Memory/1 -> unlimited RPY/2(RPY1)
  unlimited RPY/2(init) -> Memory1/1
  Memory1/1 -> unlimited RPY/3("init ")

== system manual_control_new/PX4/Acquisition ==
  motor1 : Inport
  motor2 : Inport  Port=2
  motor3 : Inport  Port=3
  motor4 : Inport  Port=4
  sensors : Inport  Port=5
  state_estim : Inport  Port=6
  MATLAB Function : MATLAB Function  TreatAsAtomicUnit=on
  Mux : Mux  Inputs=11
  DataOut : Outport
  wires:
  state_estim/1 -> MATLAB Function/1(u)
  motor1/1 -> Mux/1
  motor2/1 -> Mux/2
  motor3/1 -> Mux/3
  motor4/1 -> Mux/4
  sensors/1 -> Mux/5
  MATLAB Function/1(y1) -> Mux/6
  MATLAB Function/2(y2) -> Mux/7
  MATLAB Function/3(y3) -> Mux/8
  MATLAB Function/4(y4) -> Mux/9
  MATLAB Function/5(y5) -> Mux/10
  MATLAB Function/6(y6) -> Mux/11
  Mux/1 -> DataOut/1

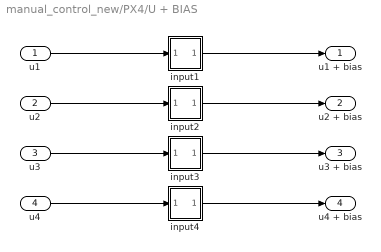
== system manual_control_new/PX4/U + BIAS ==
  u1 : Inport
  u2 : Inport  Port=2
  u3 : Inport  Port=3
  u4 : Inport  Port=4
  input1 : Subsystem
  input2 : Subsystem
  input3 : Subsystem
  input4 : Subsystem
  u1 + bias : Outport
  u2 + bias : Outport  Port=2
  u3 + bias : Outport  Port=3
  u4 + bias : Outport  Port=4
  wires:
  u2/1 -> input2/1(In1)
  u1/1 -> input1/1(In1)
  input1/1(Out1) -> u1 + bias/1
  u4/1 -> input4/1(In1)
  input4/1(Out1) -> u4 + bias/1
  input2/1(Out1) -> u2 + bias/1
  u3/1 -> input3/1(In1)
  input3/1(Out1) -> u3 + bias/1

== system manual_control_new/Observer/Observer/ filter ==
  In1 : Inport
  Demux6 : Demux  Outputs=3
  Discrete Transfer Fcn : DiscreteTransferFcn  Numerator=[Ts_slk*p]  Denominator=[1 (Ts_slk*p-1)]  SampleTime=Ts_slk
  Discrete Transfer Fcn1 : DiscreteTransferFcn  Numerator=[Ts_slk*p]  Denominator=[1 (Ts_slk*p-1)]  SampleTime=Ts_slk
  Discrete Transfer Fcn2 : DiscreteTransferFcn  Numerator=[Ts_slk*p]  Denominator=[1 (Ts_slk*p-1)]  SampleTime=Ts_slk
  Mux : Mux  Inputs=3
  Transfer Fcn1 : TransferFcn  Commented=on  Denominator=[1/p 1]
  Transfer Fcn3 : TransferFcn  Commented=on  Denominator=[1/p 1]
  Transfer Fcn4 : TransferFcn  Commented=on  Denominator=[1/p 1]
  Out1 : Outport
  wires:
  Discrete Transfer Fcn1/1 -> Mux/2
  Demux6/3 -> Discrete Transfer Fcn2/1
  Mux/1 -> Out1/1
  Discrete Transfer Fcn2/1 -> Mux/3
  Discrete Transfer Fcn/1 -> Mux/1
  In1/1 -> Demux6/1
  Demux6/1 -> Discrete Transfer Fcn/1
  Demux6/2 -> Discrete Transfer Fcn1/1

== system manual_control_new/Observer/Observer/ filter1 ==
  In1 : Inport
  Demux6 : Demux  Outputs=3
  Discrete Transfer Fcn : DiscreteTransferFcn  Numerator=[Ts_slk*p]  Denominator=[1 (Ts_slk*p-1)]  SampleTime=Ts_slk
  Discrete Transfer Fcn1 : DiscreteTransferFcn  Numerator=[Ts_slk*p]  Denominator=[1 (Ts_slk*p-1)]  SampleTime=Ts_slk
  Discrete Transfer Fcn2 : DiscreteTransferFcn  Numerator=[Ts_slk*p]  Denominator=[1 (Ts_slk*p-1)]  SampleTime=Ts_slk
  Mux : Mux  Inputs=3
  Transfer Fcn1 : TransferFcn  Commented=on  Denominator=[1/p 1]
  Transfer Fcn3 : TransferFcn  Commented=on  Denominator=[1/p 1]
  Transfer Fcn4 : TransferFcn  Commented=on  Denominator=[1/p 1]
  Out1 : Outport
  wires:
  Discrete Transfer Fcn1/1 -> Mux/2
  Demux6/3 -> Discrete Transfer Fcn2/1
  Mux/1 -> Out1/1
  Discrete Transfer Fcn2/1 -> Mux/3
  Discrete Transfer Fcn/1 -> Mux/1
  In1/1 -> Demux6/1
  Demux6/1 -> Discrete Transfer Fcn/1
  Demux6/2 -> Discrete Transfer Fcn1/1

== system manual_control_new/Observer/Observer/ filter2 ==
  In1 : Inport
  Demux6 : Demux  Outputs=3
  Discrete Transfer Fcn : DiscreteTransferFcn  Numerator=[Ts_slk*p]  Denominator=[1 (Ts_slk*p-1)]  SampleTime=Ts_slk
  Discrete Transfer Fcn1 : DiscreteTransferFcn  Numerator=[Ts_slk*p]  Denominator=[1 (Ts_slk*p-1)]  SampleTime=Ts_slk
  Discrete Transfer Fcn2 : DiscreteTransferFcn  Numerator=[Ts_slk*p]  Denominator=[1 (Ts_slk*p-1)]  SampleTime=Ts_slk
  Mux : Mux  Inputs=3
  Transfer Fcn1 : TransferFcn  Commented=on  Denominator=[1/p 1]
  Transfer Fcn3 : TransferFcn  Commented=on  Denominator=[1/p 1]
  Transfer Fcn4 : TransferFcn  Commented=on  Denominator=[1/p 1]
  Out1 : Outport
  wires:
  Discrete Transfer Fcn1/1 -> Mux/2
  Demux6/3 -> Discrete Transfer Fcn2/1
  Mux/1 -> Out1/1
  Discrete Transfer Fcn2/1 -> Mux/3
  Discrete Transfer Fcn/1 -> Mux/1
  In1/1 -> Demux6/1
  Demux6/1 -> Discrete Transfer Fcn/1
  Demux6/2 -> Discrete Transfer Fcn1/1

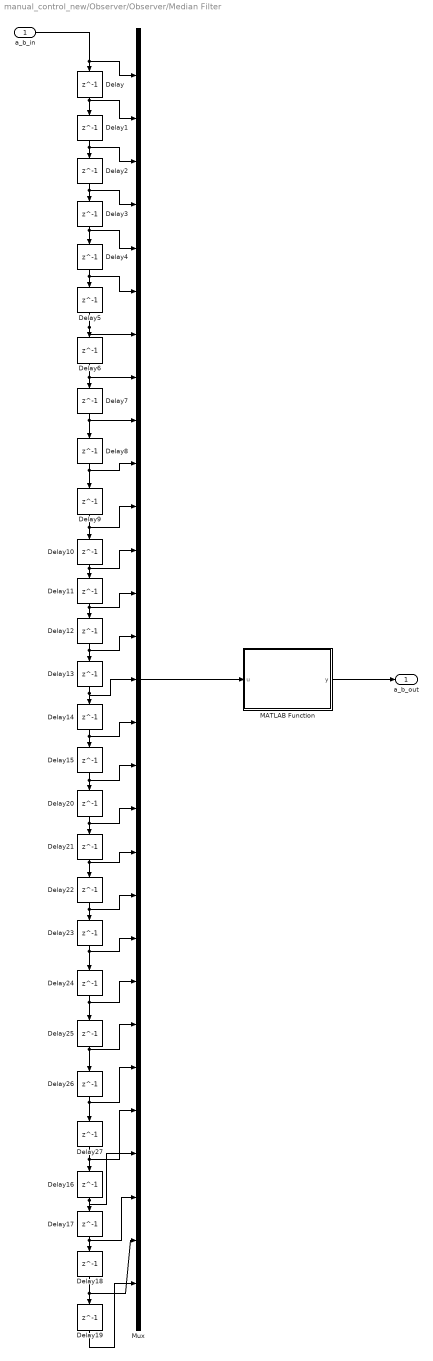
== system manual_control_new/Observer/Observer/Median Filter ==
  a_b_in : Inport
  Delay{,1..27} (28 alike) : Delay  DelayLength=1  InitialCondition=zeros(1,3)  SampleTime=Ts_slk
  MATLAB Function : MATLAB Function  TreatAsAtomicUnit=on
  Mux : Mux  Inputs=29
  a_b_out : Outport
  wires:
  a_b_in/1 -> Delay/1, Mux/1
  Delay1/1 -> Delay2/1, Mux/3
  Delay2/1 -> Delay3/1, Mux/4
  Delay/1 -> Delay1/1, Mux/2
  Delay3/1 -> Delay4/1, Mux/5
  Mux/1 -> MATLAB Function/1(u)
  MATLAB Function/1(y) -> a_b_out/1
  Delay4/1 -> Delay5/1, Mux/6
  Delay5/1 -> Delay6/1, Mux/7
  Delay6/1 -> Delay7/1, Mux/8
  Delay8/1 -> Mux/10, Delay9/1
  Delay11/1 -> Mux/13, Delay12/1
  Delay12/1 -> Mux/14, Delay13/1
  Delay7/1 -> Mux/9, Delay8/1
  Delay9/1 -> Delay10/1, Mux/11
  Delay10/1 -> Mux/12, Delay11/1
  Delay13/1 -> Mux/15, Delay14/1
  Delay24/1 -> Mux/22, Delay25/1
  Delay23/1 -> Mux/21, Delay24/1
  Delay20/1 -> Mux/18, Delay21/1
  Delay15/1 -> Mux/17, Delay20/1
  Delay21/1 -> Mux/19, Delay22/1
  Delay27/1 -> Mux/25, Delay16/1
  Delay18/1 -> Delay19/1, Mux/28
  Delay25/1 -> Mux/23, Delay26/1
  Delay22/1 -> Mux/20, Delay23/1
  Delay26/1 -> Mux/24, Delay27/1
  Delay14/1 -> Mux/16, Delay15/1
  Delay17/1 -> Mux/27, Delay18/1
  Delay16/1 -> Mux/26, Delay17/1
  Delay19/1 -> Mux/29

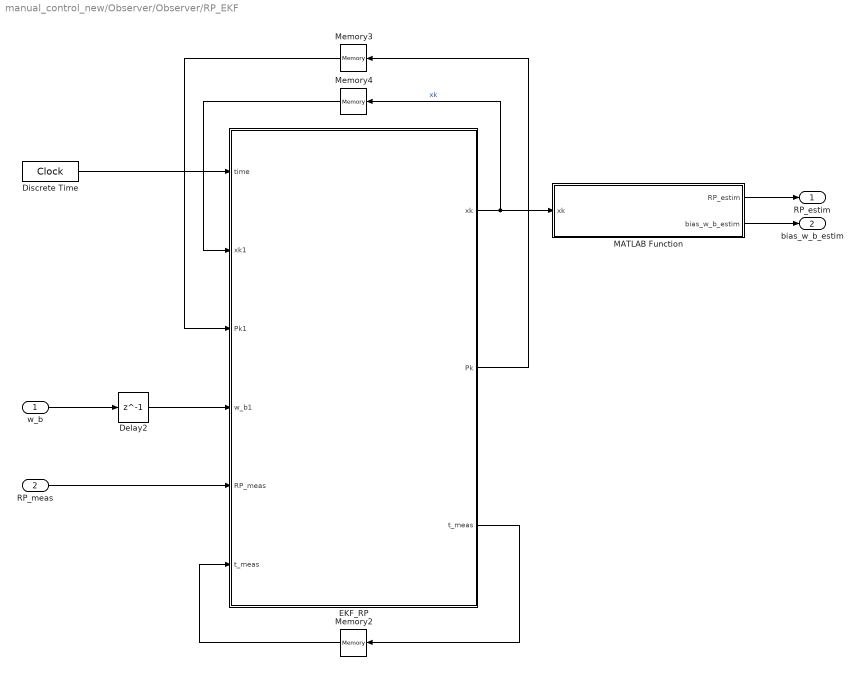
== system manual_control_new/Observer/Observer/RP_EKF ==
  w_b : Inport
  RP_meas : Inport  Port=2
  Delay2 : Delay  DelayLength=1  SampleTime=Ts_EKF_meas
  Discrete Time : DigitalClock  SampleTime=Ts_slk
  EKF_RP : MATLAB Function  TreatAsAtomicUnit=on
  MATLAB Function : MATLAB Function  TreatAsAtomicUnit=on
  Memory2 : Memory
  Memory3 : Memory  InitialCondition=P0_phth
  Memory4 : Memory  InitialCondition=x0_phth
  RP_estim : Outport
  bias_w_b_estim : Outport  Port=2
  wires:
  w_b/1 -> Delay2/1
  EKF_RP/2(Pk) -> Memory3/1
  Memory2/1 -> EKF_RP/6("t_meas ")
  EKF_RP/3(t_meas) -> Memory2/1
  RP_meas/1 -> EKF_RP/5(RP_meas)
  Discrete Time/1 -> EKF_RP/1(time)
  Memory3/1 -> EKF_RP/3(Pk1)
  Delay2/1 -> EKF_RP/4(w_b1)
  Memory4/1 -> EKF_RP/2(xk1)
  EKF_RP/1(xk) -> Memory4/1, MATLAB Function/1(xk)  "xk"
  MATLAB Function/1(RP_estim) -> RP_estim/1
  MATLAB Function/2(bias_w_b_estim) -> bias_w_b_estim/1
